simulink model "REMUS_Model"  (R2019b)
settings: Solver=VariableStepAuto  StartTime=0.0  StopTime=70  RelTol=1e-3
settings Model: Creator=7385281  LastModifiedBy=7385281
settings DataIOCC: SaveOutput=off  ReturnWorkspaceOutputs=off

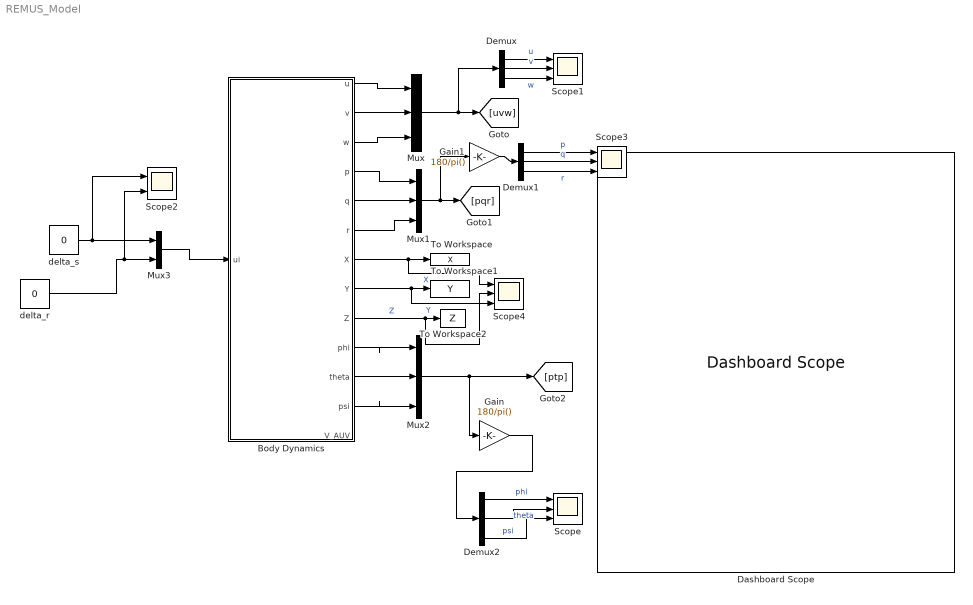
== system REMUS_Model ==
  Body Dynamics : Subsystem
  Dashboard Scope : DashboardScope
  Demux : Demux  Outputs=3
  Demux1 : Demux  Outputs=3
  Demux2 : Demux  Outputs=3
  Gain : Gain  Gain=180/pi()
  Gain1 : Gain  Gain=180/pi()
  Mux : Mux  Inputs=3
  Mux1 : Mux  Inputs=3
  Mux2 : Mux  Inputs=3
  Mux3 : Mux  Inputs=2
  Scope{,1,3..4} (4 alike) : Scope  NumInputPorts=3
  Scope2 : Scope  NumInputPorts=2
  To Workspace : ToWorkspace  VariableName=X  SampleTime=-1
      settings: Save2DSignal=2-D array (concatenate along first dimension)
  To Workspace1 : ToWorkspace  VariableName=Y  SampleTime=-1
      settings: Save2DSignal=2-D array (concatenate along first dimension)
  To Workspace2 : ToWorkspace  VariableName=Z  SampleTime=-1
      settings: Save2DSignal=2-D array (concatenate along first dimension)
  delta_r : Constant  Value=0
  delta_s : Constant  Value=0
  wires:
  Body Dynamics/2(v) -> Mux/2
  Body Dynamics/1(u) -> Mux/1
  Body Dynamics/3(w) -> Mux/3
  Mux/1 -> Demux/1, [uvw]
  Body Dynamics/4(p) -> Mux1/1
  Body Dynamics/6(r) -> Mux1/3
  Body Dynamics/5(q) -> Mux1/2
  Mux1/1 -> Gain1/1, [pqr]
  Body Dynamics/8(Y) -> Scope4/2, To Workspace1/1  "Y"
  Body Dynamics/7(X) -> Scope4/1, To Workspace/1  "X"
  Body Dynamics/9(Z) -> Scope4/3, To Workspace2/1  "Z"
  Body Dynamics/11(theta) -> Mux2/2
  Body Dynamics/10(phi) -> Mux2/1
  Body Dynamics/12(psi) -> Mux2/3
  Mux2/1 -> Gain/1, [ptp]
  Mux3/1 -> Body Dynamics/1(ui)
  delta_s/1 -> Scope2/1, Mux3/1
  delta_r/1 -> Scope2/2, Mux3/2
  Demux/1 -> Scope1/1  "u"
  Demux/2 -> Scope1/2  "v"
  Demux/3 -> Scope1/3  "w"
  Demux1/1 -> Scope3/1  "p"
  Demux1/2 -> Scope3/2  "q"
  Demux1/3 -> Scope3/3  "r"
  Demux2/1 -> Scope/1  "phi"
  Demux2/2 -> Scope/2  "theta"
  Demux2/3 -> Scope/3  "psi"
  Gain/1 -> Demux2/1
  Gain1/1 -> Demux1/1

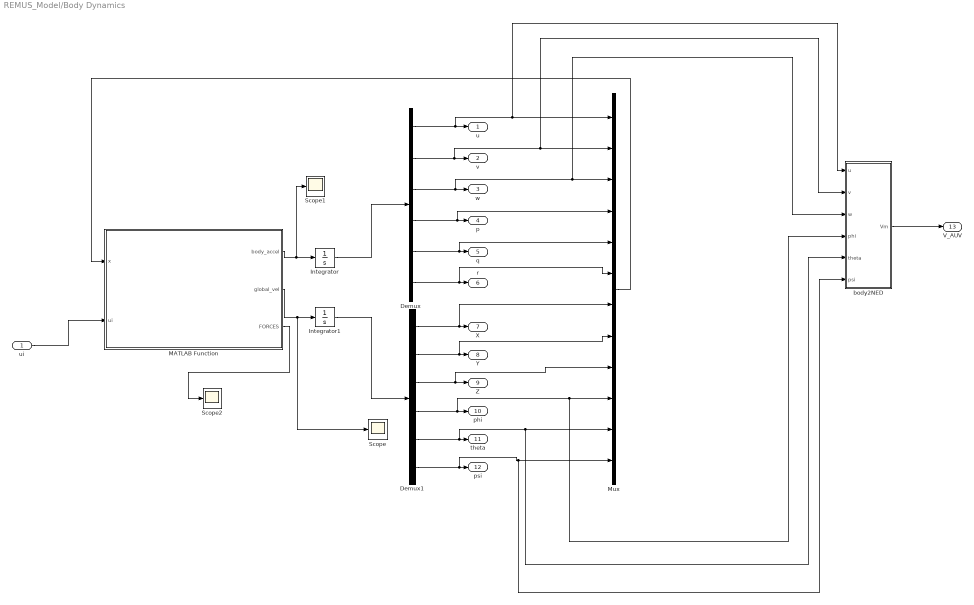
== system REMUS_Model/Body Dynamics ==
  ui : Inport
  Demux : Demux  Outputs=6
  Demux1 : Demux  Outputs=6
  Integrator : Integrator  InitialCondition=[1.54; 0 ; 0; 0; 0; 0]
  Integrator1 : Integrator  InitialCondition=[0; 0; 0.0196; -5*pi/180; 0; 0]
  MATLAB Function : MATLAB Function  TreatAsAtomicUnit=on
  Mux : Mux  Inputs=12
  Scope : Scope
  Scope1 : Scope
  Scope2 : Scope
  body2NED : MATLAB Function  TreatAsAtomicUnit=on
  u : Outport
  v : Outport  Port=2
  w : Outport  Port=3
  p : Outport  Port=4
  q : Outport  Port=5
  r : Outport  Port=6
  X : Outport  Port=7
  Y : Outport  Port=8
  Z : Outport  Port=9
  phi : Outport  Port=10
  theta : Outport  Port=11
  psi : Outport  Port=12
  V_AUV : Outport  Port=13
  wires:
  Integrator/1 -> Demux/1
  Demux/5 -> Mux/5, q/1
  MATLAB Function/1(body_accel) -> Scope1/1, Integrator/1
  Demux/1 -> Mux/1, body2NED/1(u), u/1
  Demux/6 -> Mux/6, r/1
  Demux/2 -> Mux/2, body2NED/2(v), v/1
  Demux/3 -> body2NED/3(w), Mux/3, w/1
  Demux/4 -> Mux/4, p/1
  ui/1 -> MATLAB Function/2(ui)
  Integrator1/1 -> Demux1/1
  Demux1/6 -> body2NED/6(psi), Mux/12, psi/1
  Demux1/1 -> Mux/7, X/1
  Demux1/3 -> Mux/9, Z/1
  Demux1/5 -> body2NED/5(theta), Mux/11, theta/1
  Demux1/2 -> Mux/8, Y/1
  Mux/1 -> MATLAB Function/1(x)
  Demux1/4 -> body2NED/4(phi), Mux/10, phi/1
  body2NED/1(Vm) -> V_AUV/1
  MATLAB Function/2(global_vel) -> Scope/1, Integrator1/1
  MATLAB Function/3(FORCES) -> Scope2/1

== matlab function REMUS_Model/Body Dynamics/MATLAB Function ==
  data: x input; body_accel output; ui input; global_vel output; FORCES output
% REMUS.M Vehicle Simulator, returns the 
%   time derivative of the state vector
function [body_accel,global_vel,FORCES] = remus(x,ui)
% TERMS
% ---------------------------------------------------------------------
% STATE VECTOR:
% x = [u v w p q r xpos ypos zpos phi theta psi]'
% Body-referenced Coordinates
% u = Surge velocity [m/sec]
% v = Sway velocity [m/sec]
% w = Heave velocity [m/sec]
% p = Roll rate [rad/sec]
% q = Pitch rate [rad/sec]
% r = Yaw rate [rad/sec]
% Earth-fixed coordinates
% xpos = Position in x-direction [m]
% ypos = Position in y-direction [m]
% zpos = Position in z-direction [m]
% phi = Roll angle [rad]
% theta = Pitch angle [rad]
% psi = Yaw angle [rad]
% INPUT VECTOR
% ui = [delta_s delta_r]'
% Control Fin Angles
% delta-s = angle of stern planes [rad]
% delta-r = angle of rudder planes [rad]
% Initialize global variables
%7---------------------------------------------------------------------

% -------------------------------------------------------------------------
% Vehicle Parameters:
% -------------------------------------------------------------------------
m = 30.4791; % mass [kg]
W = +2.99e+002;% Measured Vehicle Weight [N]
B = +3.08e+002;  % Measured Vehicle Bouynacy  [N]
delta_max = 30*pi/180; % Max deflection of control input

% -------------------------------------------------------------------------
% Table A.3: Center of Buoyancy wrt Origin at Vehicle Nose
% -------------------------------------------------------------------------
xb = -6.11e-001; %[m]
yb = +0.00e+000; %[m]
zb = +0.00e+000; %[m]

% -------------------------------------------------------------------------
% Table A.4: Center of Gravity wrt Origin at CB
% -------------------------------------------------------------------------
xg = +0.00e+000; % m
yg = +0.00e+000; % m
zg = +1.96e-002;% m

Ixx = 0.1770; % Inertia about x-axis [kg*m^2]
Iyy = 3.4500; % Inertia about y-axis [kg*m^2]
Izz = 3.4500; % Inertia about z-axis [kg*m^2]

% -------------------------------------------------------------------------
% Axial Drag Coefficient
% -------------------------------------------------------------------------
Xuu = -1.62e+000; %[kg/m]

% -------------------------------------------------------------------------
% Table C.2: Crossflow Drag Coefficients
% -------------------------------------------------------------------------
Yvv = -1.31e+003; % kg/m
Yrr = +6.32e-001; % kg -m/rad 
Zww = -1.31e+002; % kg/m 
Zqq = -6.32e-001; % kg m/rad2
Mwwd = +3.18e+000; % kg 
Mqq = -1.88e+002; % kg m2/rad
Nvvd = -3.18e+000; % kg
Nrr = -9.40e+001; % kg.m2/rad 2

% -------------------------------------------------------------------------
% Table C.3: Rolling Resistance Coefficient
% -------------------------------------------------------------------------
Kpp = -1.30e-001; % kg-m2/rad'

% -------------------------------------------------------------------------
% Table C.4: Body Lift and Moment Coefficients
% -------------------------------------------------------------------------
Yuv = -2.86e+001; % kg/m 
Zuw = -2.86e+001; % kg/m
Muwb = -4.47e+000; % kg
Nuvb = +4.47e+000; % kg
  

% -------------------------------------------------------------------------
% Table C.5: Added Mass Coefficients
% -------------------------------------------------------------------------
Xudot = -9.30e-001 ; % kg
Yvdot = -3.55e+001 ; % kg
Yrdot = +1.93e+000 ; % kg. m/rad
Zwdot = -3.55e+001 ; % kg
Zqdot = -1.93e+000 ; % kg. m/rad
Kpdot = -7.04e-002 ; % kg-m2 /rad
Mwdot = -1.93e+000 ; % kg. m  
Mqdot = -4.88e+000 ; % kg-m2 /rad
Nvdot = +1.93e+000 ; % kg-m
Nrdot = -4.88e+000 ; % kg-m2 /rad

% -------------------------------------------------------------------------
% Table C.6: Added Mass Force Cross-term Coefficients
% -------------------------------------------------------------------------
Xwq = -3.55e+001 ; % kg/rad
Xqq = -1.93e+000 ; % kg-m/rad
Xvr = +3.55e+001 ; % kg/rad
Xrr = -1.93e+000 ; % kg m/rad
Yura= -9.30e-001 ; % kg/rad
Ywp = +3.55e+001 ; % kg/rad
Ypq = +1.93e+000 ; % kg m/rad
Zuqa= +9.30e-001 ; % kg/rad
Zvp = -3.55e+001 ; % kg/rad
Zrp = +1.93e+000 ; % kg/rad

% -------------------------------------------------------------------------
% Table C.7: Added Mass K-Moment Cross-term Coefficients
% -------------------------------------------------------------------------
% ALL Zero 

% -------------------------------------------------------------------------
% Table C.8: Added Mass M-, N-Moment Cross-term Coefficients
% -------------------------------------------------------------------------
Muqa = +1.93e+000 ; % kg m/rad
Muwa = +3.46e+001  ; % kg
Mvp  = -1.93e+000 ; % kg-m/rad
Mrp  = +4.86e+000  ; % kg-m2/rad2
Nuva = -3.46e+001  ; % kg
Nura = +1.93e+000 ; % kg- m/rad
Nwp  = -1.93e+000  ; % kg- m/rad
Npq  = -4.86e+000  ; % kg- m2/rad2

% -------------------------------------------------------------------------
% Table C.9: Propeller Terms
% -------------------------------------------------------------------------
Xprop = +3.86e+000; % N
%Xprop = 15;
Kprop = -5.43e-001; % N-m


% -------------------------------------------------------------------------
% Table C.10: Table C.10: Control Fin Coefficients
% -------------------------------------------------------------------------

Yuudr = +9.64e+000 ; % kg/(m- rad)
Zuuds = -9.64e+000 ; % kg/(m- rad)
Muuds = -6.15e+000 ; % kg/rad
Nuudr = -6.15e+000 ; % kg/rad
Yuvf  = -9.64e+000 ; % kg/m
Zuwf  = -9.64e+000 ; % kg/m
Yurf  = +6.15e+000 ; % kg/rad
Zuqf  = -6.15e+000 ; % kg/rad
Muwf  = -6.15e+000 ; % kg
Nuvf  = +6.15e+000 ; % kg
Muqf  = -3.93e+000 ; % kg m/rad
Nurf  = -3.93e+000 ; % kg m/rad

% Missing Terms 
% ---------------------------------------------------------------------
% Table B.1: Non-Linear Force Coefficients
% ---------------------------------------------------------------------
Yur = Yura + Yurf; % Kg/rad Added Mass Cross Term and Fin Lift
Zuq = Zuqa + Zuqf; % Kg/rad Added Mass Cross Term and Fin Lift
Mww = Mwwd;
Nvv = Nvvd;
Muq = Muqa + Muqf;
Muw = Muwa + Muwf;
Nuv = Nuva + Nuvf; 
Nur = Nura + Nurf;


Minv = zeros(6,6);
Minv = [m-Xudot 0 0 0 m*zg -m*yg;...
    0 m-Yvdot 0 -m*zg 0 m*xg-Yrdot;...
    0 0 m-Zwdot m*yg -m*xg-Zqdot 0;...
    0 -m*zg m*yg Ixx-Kpdot 0 0;...
    m*zg 0 -m*xg-Mwdot 0 Iyy-Mqdot 0;...
    -m*yg m*xg-Nvdot 0 0 0 Izz-Nrdot]^-1;

% Output flags
% show_forces = 10;
% Get and check state variables and control inputs
% Get state variables
u =x(1); 
v =x(2); 
w =x(3); 
p =x(4); 
q = x(5);
r = x(6); 
phi = x(10); 
theta = x(11); 
psi = x(12);

% Get control inputs
delta_s = ui(1); delta_r = ui(2);

% Check control inputs (useful later)
if delta_s > delta_max
delta_s = sign(delta_s)*delta_max;
end
if delta_r > delta_max   % This may cause issue - Ben C.
delta_r = sign(delta_r)*delta_max;
end

% Initialize elements of coordinate system transform matrix
%--------------------------------------------------------------------------
c1 = cos(phi);
c2 = cos(theta);
c3 = cos(psi);
s1 = sin(phi); 
s2 =sin(theta); 
s3 = sin(psi); 
t2 = tan(theta);

% Set total forces from equations of motion
%--------------------------------------------------------------------------

X = -(W-B)*sin(theta) + Xuu*u*abs(u) + (Xwq-m)*w*q + (Xqq +m*xg)*q^2 ...
+ (Xvr+m)*v*r + (Xrr + m*xg)*r^2 -m*yg*p*q - m*zg*p*r ...
+ Xprop;

Y = (W-B)*cos(theta)*sin(phi) + Yvv*v*abs(v) + Yrr*r*abs(r) +Yuv*u*v ...
+ (Ywp+m)*w*p + (Yur-m)*u*r - (m*zg)*q*r + (Ypq - m*xg)*p*q ...
+ Yuudr*u^2*delta_r;

Z = (W-B)*cos(theta)*cos(phi) + Zww*w*abs(w) + Zqq*q*abs(q)+Zuw*u*w ...
+ (Zuq+m)*u*q + (Zvp-m)*v*p + (m*zg)*p^2 + (m*zg)*q^2 ...
+ (Zrp - m*xg)*r*p + Zuuds*u^2*delta_s;

K = -(yg*W-yb*B)*cos(theta)*cos(phi) -(zg*W-zb*B)*cos(theta)*sin(phi) ...
+ Kpp*p*abs(p) - (Izz-Iyy)*q*r - (m*zg)*w*p + (m*zg)*u*r + Kprop;

M = -(zg*W-zb*B)*sin(theta) - (xg*W-xb*B)*cos(theta)*cos(phi) +Mww*w*abs(w) ...
+ Mqq*q*abs(q) + (Mrp - (Ixx-Izz))*r*p + (m*zg)*v*r - (m*zg)*w*q ...
+ (Muq - m*xg)*u*q + Muw*u*w + (Mvp + m*xg)*v*p ...
+ Muuds*u^2*delta_s;

N = -(xg*W-xb*B)*cos(theta)*sin(phi) - (yg*W-yb*B)*sin(theta) ...
+ Nvv*v*abs(v) + Nrr*r*abs(r) + Nuv*u*v ...
+ (Npq - (Iyy-Ixx))*p*q + (Nwp - m*xg)*w*p + (Nur + m*xg)*u*r ...
+ Nuudr*u^2*delta_r ;

N = 0;

K = 0;
M = 0;
FORCES = [X Y Z K M N]';

% Body Fixed Accelerations [udot vdot wdot pdot qdot rdot]'
%{
body_accel =...
[Minv(1,1)*X+Minv(1,2)*Y+Minv(1,3)*Z+Minv(1,4)*K+Minv(1,5)*M+Minv(1,6)*N;...
Minv(2,1)*X+Minv(2,2)*Y+Minv(2,3)*Z+Minv(2,4)*K+Minv(2,5)*M+Minv(2,6)*N;...
Minv(3,1)*X+Minv(3,2)*Y+Minv(3,3)*Z+Minv(3,4)*K+Minv(3,5)*M+Minv(3,6)*N;...
Minv(4,1)*X+Minv(4,2)*Y+Minv(4,3)*Z+Minv(4,4)*K+Minv(4,5)*M+Minv(4,6)*N;...
Minv(5,1)*X+Minv(5,2)*Y+Minv(5,3)*Z+Minv(5,4)*K+Minv(5,5)*M+Minv(5,6)*N;...
Minv(6,1)*X+Minv(6,2)*Y+Minv(6,3)*Z+Minv(6,4)*K+Minv(6,5)*M+Minv(6,6)*N];
%}
body_accel = Minv*FORCES;
% Global Velocities [xdot ydot zdot phidot thetadot psidot]'
global_vel=[c3*c2*u+(c3*s2*s1-s3*c1)*v+(s3*s1+c3*c1*s2)*w;...
s3*c2*u+(c1*c3+s1*s2*s3)*v+(c1*s2*s3-c3*s1)*w;...
-s2*u+c2*s1*v+c1*c2*w;...
p+s1*t2*q+c1*t2*r;...
c1*q-s1*r;...
s1/c2*q+c1/c2*r];

== matlab function REMUS_Model/Body Dynamics/body2NED ==
  data: u input; v input; w input; phi input; theta input; psi input; Vm output
function Vm= fcn(u,v,w,phi,theta,psi)
N=[cos(theta)*cos(psi) (sin(phi)*sin(theta)*cos(psi)-cos(phi)*sin(psi)) (cos(phi)*sin(theta)*cos(psi)+sin(phi)*sin(psi));
   -cos(theta)*sin(psi) -(sin(phi)*sin(theta)*sin(psi)+cos(phi)*cos(psi)) -(cos(phi)*sin(theta)*sin(psi) - sin(phi)*cos(psi));
   sin(theta) -sin(phi)*cos(theta) -cos(phi)*cos(theta)];
Vm=N*[u;v;w];
end
